simulink subsystem "Vehiculo"  (R2023b)
settings: Solver=VariableStepAuto  StartTime=0.0  StopTime=10.0  RelTol=1e-3
settings Model: Creator=pablo  LastModifiedBy=pablo

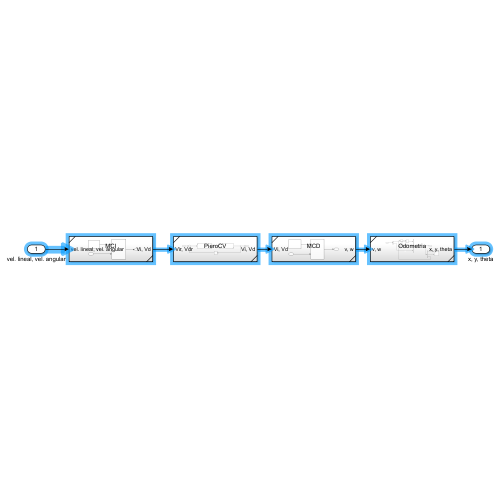
[thumbnail: Simulink's stored preview of the top-level diagram]
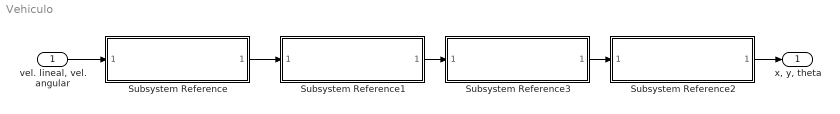
== system Vehiculo ==
  "vel. lineal, vel. angular" : Inport
  Subsystem Reference : Subsystem  ReferencedSubsystem=MCI
  Subsystem Reference1 : Subsystem  ReferencedSubsystem=PieroCV
  Subsystem Reference2 : Subsystem  ReferencedSubsystem=Odometria
  Subsystem Reference3 : Subsystem  ReferencedSubsystem=MCD
  "x, y, theta" : Outport
  wires:
  Subsystem Reference/1 -> Subsystem Reference1/1
  Subsystem Reference3/1 -> Subsystem Reference2/1
  Subsystem Reference1/1 -> Subsystem Reference3/1
  Subsystem Reference2/1 -> "x, y, theta"/1
  "vel. lineal, vel. angular"/1 -> Subsystem Reference/1
